simulink model "HelicopterSystem"  (R2019b)
settings: Solver=VariableStepAuto  StartTime=0.0  StopTime=10.0  RelTol=1e-3
settings Model: DataDictionary=HeliSystemDD.sldd  Creator=bpotter  LastModifiedBy=bpotter
settings DataIOCC: ExternalInput=input  LoadExternalInput=on  SaveOutput=off  DSMLogging=off  SaveTime=off  ReturnWorkspaceOutputs=off
settings OptimizationCC: UseDivisionForNetSlopeComputation=on
settings SFSimCC: CustomCodeUndefinedFunction=UseInterfaceOnly
settings ConfigComp: CovScope=ReferencedModels  CovIncludeTopModel=off

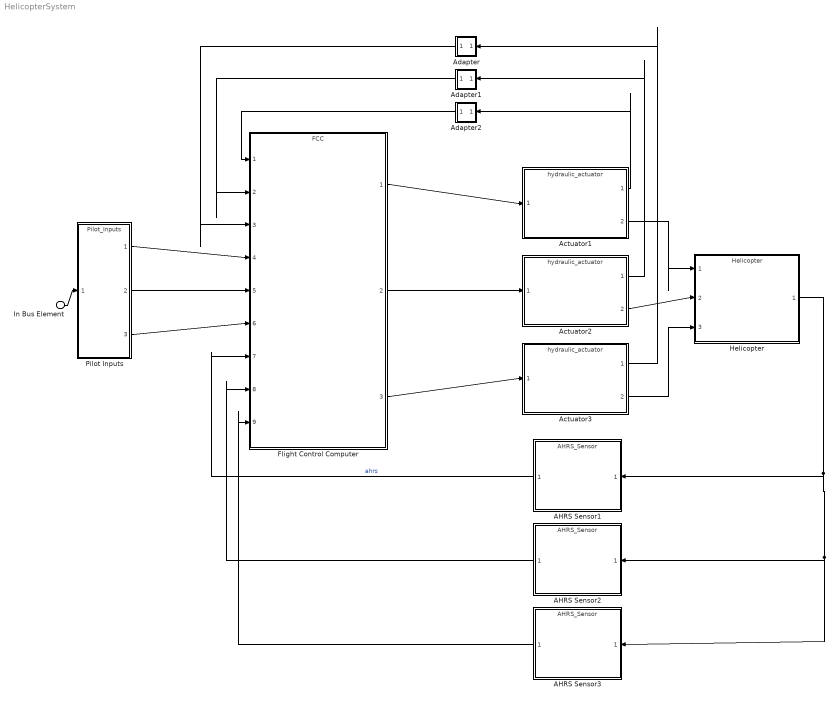
== system HelicopterSystem ==
  In Bus Element : Inport  PortName=Pilot
  "AHRS Sensor1  " : ModelReference  ModelNameDialog=AHRS_Sensor  SimulationMode=Normal  ModelReferenceVersion=1.170
      settings: PortSchema="{\"entries\":[{\"content\":{\"headerSize\":38,\"margin\":15,\"minimumSpacing\":25,\"sides\":[{\"content\":{\"connectorIds\":[\"Out1\"]},\"type\":\"ConnectorPlacement.EquallySpacedRectSide\",\"uuid\":\"b92c4a61-dac7-4e8b-978a-518464efd6dc\"},{\"content\":{\"connectorIds\":[\"In1\"],\"side\":\"RIGHT\"},\"type\":\"ConnectorPlacement.EquallySpacedRectSide\",\"uuid\":\"7fdd65f0-967d-4e66-9e23-32118f2eba6a\"},{\"content\":{\"connectorIds\":[],\"side\":\"TOP\"},\"type\":\"ConnectorPlacement.EquallySpacedRectSide\",\"uuid\":\"3746c468-edd5-479d-86e4-82fa38f92dc3\"},{\"content\":{\"connectorIds\":[],\"side\":\"BOTTOM\"},\"type\":\"ConnectorPlacement.EquallySpacedRectSide\",\"uuid\":\"6d40d3fe-09a5-49bd-a6ff-4bc99f24213d\"}]},\"type\":\"ConnectorPlacement.EquallySpacedConnector\",\"uuid\":\"540cabe7-683b-4658-aa3c-75031e0ce477\"}],\"packageUris\":[\"http:\\/\\/schema.mathworks.com\\/mf0\\/Connector\\/19700101\"],\"version\":\"1.0\"}"
  AHRS Sensor2 : ModelReference  ModelNameDialog=AHRS_Sensor  SimulationMode=Normal  ModelReferenceVersion=1.170
      settings: PortSchema="{\"entries\":[{\"content\":{\"headerSize\":38,\"margin\":15,\"minimumSpacing\":25,\"sides\":[{\"content\":{\"connectorIds\":[\"Out1\"]},\"type\":\"ConnectorPlacement.EquallySpacedRectSide\",\"uuid\":\"b92c4a61-dac7-4e8b-978a-518464efd6dc\"},{\"content\":{\"connectorIds\":[\"In1\"],\"side\":\"RIGHT\"},\"type\":\"ConnectorPlacement.EquallySpacedRectSide\",\"uuid\":\"7fdd65f0-967d-4e66-9e23-32118f2eba6a\"},{\"content\":{\"connectorIds\":[],\"side\":\"TOP\"},\"type\":\"ConnectorPlacement.EquallySpacedRectSide\",\"uuid\":\"3746c468-edd5-479d-86e4-82fa38f92dc3\"},{\"content\":{\"connectorIds\":[],\"side\":\"BOTTOM\"},\"type\":\"ConnectorPlacement.EquallySpacedRectSide\",\"uuid\":\"e1e7bc22-7c0e-4a7f-891e-467da093d39e\"}]},\"type\":\"ConnectorPlacement.EquallySpacedConnector\",\"uuid\":\"540cabe7-683b-4658-aa3c-75031e0ce477\"}],\"packageUris\":[\"http:\\/\\/schema.mathworks.com\\/mf0\\/Connector\\/19700101\"],\"version\":\"1.0\"}"
  AHRS Sensor3 : ModelReference  ModelNameDialog=AHRS_Sensor  SimulationMode=Normal  ModelReferenceVersion=1.170
      settings: PortSchema="{\"entries\":[{\"content\":{\"headerSize\":38,\"margin\":15,\"minimumSpacing\":25,\"sides\":[{\"content\":{\"connectorIds\":[\"Out1\"]},\"type\":\"ConnectorPlacement.EquallySpacedRectSide\",\"uuid\":\"b92c4a61-dac7-4e8b-978a-518464efd6dc\"},{\"content\":{\"connectorIds\":[\"In1\"],\"side\":\"RIGHT\"},\"type\":\"ConnectorPlacement.EquallySpacedRectSide\",\"uuid\":\"7fdd65f0-967d-4e66-9e23-32118f2eba6a\"},{\"content\":{\"connectorIds\":[],\"side\":\"TOP\"},\"type\":\"ConnectorPlacement.EquallySpacedRectSide\",\"uuid\":\"3746c468-edd5-479d-86e4-82fa38f92dc3\"},{\"content\":{\"connectorIds\":[],\"side\":\"BOTTOM\"},\"type\":\"ConnectorPlacement.EquallySpacedRectSide\",\"uuid\":\"265bdab0-2fd8-4d9f-89ea-736dcc13bf3d\"}]},\"type\":\"ConnectorPlacement.EquallySpacedConnector\",\"uuid\":\"540cabe7-683b-4658-aa3c-75031e0ce477\"}],\"packageUris\":[\"http:\\/\\/schema.mathworks.com\\/mf0\\/Connector\\/19700101\"],\"version\":\"1.0\"}"
  Actuator1 : ModelReference  ModelNameDialog=hydraulic_actuator  SimulationMode=Normal  ModelReferenceVersion=1.113
      settings: PortSchema="{\"entries\":[{\"content\":{\"headerSize\":38,\"margin\":15,\"minimumSpacing\":25,\"sides\":[{\"content\":{\"connectorIds\":[\"In1\"]},\"type\":\"ConnectorPlacement.EquallySpacedRectSide\",\"uuid\":\"fc9e68fb-3587-497f-b8aa-5fffad76bdc9\"},{\"content\":{\"connectorIds\":[\"Out1\",\"Out2\"],\"side\":\"RIGHT\"},\"type\":\"ConnectorPlacement.EquallySpacedRectSide\",\"uuid\":\"35b616a7-1e7e-4bab-abf4-1bdc7c33d6ef\"},{\"content\":{\"connectorIds\":[],\"side\":\"TOP\"},\"type\":\"ConnectorPlacement.EquallySpacedRectSide\",\"uuid\":\"7330c33a-79c0-425b-bf03-91b7ec739e63\"}]},\"type\":\"ConnectorPlacement.EquallySpacedConnector\",\"uuid\":\"e9501eb8-1a55-4d46-b5aa-5edf970ac40b\"}],\"packageUris\":[\"http:\\/\\/schema.mathworks.com\\/mf0\\/Connector\\/19700101\"],\"version\":\"1.0\"}"
  Actuator2 : ModelReference  ModelNameDialog=hydraulic_actuator  SimulationMode=Normal  ModelReferenceVersion=1.113
      settings: PortSchema="{\"entries\":[{\"content\":{\"headerSize\":38,\"margin\":15,\"minimumSpacing\":25,\"sides\":[{\"content\":{\"connectorIds\":[\"In1\"]},\"type\":\"ConnectorPlacement.EquallySpacedRectSide\",\"uuid\":\"fc9e68fb-3587-497f-b8aa-5fffad76bdc9\"},{\"content\":{\"connectorIds\":[\"Out1\",\"Out2\"],\"side\":\"RIGHT\"},\"type\":\"ConnectorPlacement.EquallySpacedRectSide\",\"uuid\":\"35b616a7-1e7e-4bab-abf4-1bdc7c33d6ef\"},{\"content\":{\"connectorIds\":[],\"side\":\"TOP\"},\"type\":\"ConnectorPlacement.EquallySpacedRectSide\",\"uuid\":\"7330c33a-79c0-425b-bf03-91b7ec739e63\"}]},\"type\":\"ConnectorPlacement.EquallySpacedConnector\",\"uuid\":\"e9501eb8-1a55-4d46-b5aa-5edf970ac40b\"}],\"packageUris\":[\"http:\\/\\/schema.mathworks.com\\/mf0\\/Connector\\/19700101\"],\"version\":\"1.0\"}"
  Actuator3 : ModelReference  ModelNameDialog=hydraulic_actuator  SimulationMode=Normal  ModelReferenceVersion=1.113
      settings: PortSchema="{\"entries\":[{\"content\":{\"headerSize\":38,\"margin\":15,\"minimumSpacing\":25,\"sides\":[{\"content\":{\"connectorIds\":[\"In1\"]},\"type\":\"ConnectorPlacement.EquallySpacedRectSide\",\"uuid\":\"fc9e68fb-3587-497f-b8aa-5fffad76bdc9\"},{\"content\":{\"connectorIds\":[\"Out1\",\"Out2\"],\"side\":\"RIGHT\"},\"type\":\"ConnectorPlacement.EquallySpacedRectSide\",\"uuid\":\"35b616a7-1e7e-4bab-abf4-1bdc7c33d6ef\"},{\"content\":{\"connectorIds\":[],\"side\":\"TOP\"},\"type\":\"ConnectorPlacement.EquallySpacedRectSide\",\"uuid\":\"7330c33a-79c0-425b-bf03-91b7ec739e63\"}]},\"type\":\"ConnectorPlacement.EquallySpacedConnector\",\"uuid\":\"e9501eb8-1a55-4d46-b5aa-5edf970ac40b\"}],\"packageUris\":[\"http:\\/\\/schema.mathworks.com\\/mf0\\/Connector\\/19700101\"],\"version\":\"1.0\"}"
  Adapter : Subsystem
      settings: PortSchema="{\"entries\":[{\"content\":{\"margin\":10,\"minimumSpacing\":10,\"sides\":[{\"content\":{\"connectorIds\":[\"Out1\"]},\"type\":\"ConnectorPlacement.EquallySpacedRectSide\",\"uuid\":\"3ae78bc2-40c3-4405-b1e9-aa99f01667e3\"},{\"content\":{\"connectorIds\":[\"In1\"],\"side\":\"RIGHT\"},\"type\":\"ConnectorPlacement.EquallySpacedRectSide\",\"uuid\":\"ba8b0a16-3184-49c7-8dc0-2ecd07e7bfdb\"},{\"content\":{\"connectorIds\":[],\"side\":\"TOP\"},\"type\":\"ConnectorPlacement.EquallySpacedRectSide\",\"uuid\":\"2e1b4a4d-beaa-4cad-b3d0-913db021f2bf\"},{\"content\":{\"connectorIds\":[],\"side\":\"BOTTOM\"},\"type\":\"ConnectorPlacement.EquallySpacedRectSide\",\"uuid\":\"ce88d55a-ed5b-4e72-9847-8844dc7d3e9c\"}]},\"type\":\"ConnectorPlacement.EquallySpacedConnector\",\"uuid\":\"3893b0a5-5763-428c-b0ac-b513abbdb3d9\"}],\"packageUris\":[\"http://schema.mathworks.com/mf0/Connector/19700101\"],\"version\":\"1.0\"}"
  Adapter1 : Subsystem
      settings: PortSchema="{\"entries\":[{\"content\":{\"margin\":10,\"minimumSpacing\":10,\"sides\":[{\"content\":{\"connectorIds\":[\"Out1\"]},\"type\":\"ConnectorPlacement.EquallySpacedRectSide\",\"uuid\":\"3ae78bc2-40c3-4405-b1e9-aa99f01667e3\"},{\"content\":{\"connectorIds\":[\"In1\"],\"side\":\"RIGHT\"},\"type\":\"ConnectorPlacement.EquallySpacedRectSide\",\"uuid\":\"ba8b0a16-3184-49c7-8dc0-2ecd07e7bfdb\"},{\"content\":{\"connectorIds\":[],\"side\":\"TOP\"},\"type\":\"ConnectorPlacement.EquallySpacedRectSide\",\"uuid\":\"2e1b4a4d-beaa-4cad-b3d0-913db021f2bf\"},{\"content\":{\"connectorIds\":[],\"side\":\"BOTTOM\"},\"type\":\"ConnectorPlacement.EquallySpacedRectSide\",\"uuid\":\"ce88d55a-ed5b-4e72-9847-8844dc7d3e9c\"}]},\"type\":\"ConnectorPlacement.EquallySpacedConnector\",\"uuid\":\"3893b0a5-5763-428c-b0ac-b513abbdb3d9\"}],\"packageUris\":[\"http://schema.mathworks.com/mf0/Connector/19700101\"],\"version\":\"1.0\"}"
  Adapter2 : Subsystem
      settings: PortSchema="{\"entries\":[{\"content\":{\"margin\":10,\"minimumSpacing\":10,\"sides\":[{\"content\":{\"connectorIds\":[\"Out1\"]},\"type\":\"ConnectorPlacement.EquallySpacedRectSide\",\"uuid\":\"3ae78bc2-40c3-4405-b1e9-aa99f01667e3\"},{\"content\":{\"connectorIds\":[\"In1\"],\"side\":\"RIGHT\"},\"type\":\"ConnectorPlacement.EquallySpacedRectSide\",\"uuid\":\"ba8b0a16-3184-49c7-8dc0-2ecd07e7bfdb\"},{\"content\":{\"connectorIds\":[],\"side\":\"TOP\"},\"type\":\"ConnectorPlacement.EquallySpacedRectSide\",\"uuid\":\"2e1b4a4d-beaa-4cad-b3d0-913db021f2bf\"},{\"content\":{\"connectorIds\":[],\"side\":\"BOTTOM\"},\"type\":\"ConnectorPlacement.EquallySpacedRectSide\",\"uuid\":\"ce88d55a-ed5b-4e72-9847-8844dc7d3e9c\"}]},\"type\":\"ConnectorPlacement.EquallySpacedConnector\",\"uuid\":\"3893b0a5-5763-428c-b0ac-b513abbdb3d9\"}],\"packageUris\":[\"http://schema.mathworks.com/mf0/Connector/19700101\"],\"version\":\"1.0\"}"
  Flight Control Computer : ModelReference  ModelNameDialog=FCC  SimulationMode=Normal  ModelReferenceVersion=1.70
      settings: PortSchema="{\"entries\":[{\"content\":{\"headerSize\":38,\"margin\":15,\"minimumSpacing\":25,\"sides\":[{\"content\":{\"connectorIds\":[\"In1\",\"In2\",\"In3\",\"In4\",\"In5\",\"In6\",\"In7\",\"In8\",\"In9\"]},\"type\":\"ConnectorPlacement.EquallySpacedRectSide\",\"uuid\":\"9959663a-a09f-47a8-9233-f49ef842a145\"},{\"content\":{\"connectorIds\":[\"Out1\",\"Out2\",\"Out3\"],\"side\":\"RIGHT\"},\"type\":\"ConnectorPlacement.EquallySpacedRectSide\",\"uuid\":\"4d21989f-a787-4fcb-862b-70f89eaf4b18\"},{\"content\":{\"connectorIds\":[],\"side\":\"TOP\"},\"type\":\"ConnectorPlacement.EquallySpacedRectSide\",\"uuid\":\"c2e05887-1556-4bab-9344-e41638b7e6c9\"}]},\"type\":\"ConnectorPlacement.EquallySpacedConnector\",\"uuid\":\"3e276280-9190-46ce-8e07-322db49b607e\"}],\"packageUris\":[\"http:\\/\\/schema.mathworks.com\\/mf0\\/Connector\\/19700101\"],\"version\":\"1.0\"}"
  Helicopter : ModelReference  ModelNameDialog=Helicopter  SimulationMode=Normal  ModelReferenceVersion=1.168
      settings: PortSchema="{\"entries\":[{\"content\":{\"headerSize\":38,\"margin\":15,\"minimumSpacing\":25,\"sides\":[{\"content\":{\"connectorIds\":[\"In1\",\"In2\",\"In3\"]},\"type\":\"ConnectorPlacement.EquallySpacedRectSide\",\"uuid\":\"b92c4a61-dac7-4e8b-978a-518464efd6dc\"},{\"content\":{\"connectorIds\":[\"Out1\"],\"side\":\"RIGHT\"},\"type\":\"ConnectorPlacement.EquallySpacedRectSide\",\"uuid\":\"7fdd65f0-967d-4e66-9e23-32118f2eba6a\"},{\"content\":{\"connectorIds\":[],\"side\":\"TOP\"},\"type\":\"ConnectorPlacement.EquallySpacedRectSide\",\"uuid\":\"3746c468-edd5-479d-86e4-82fa38f92dc3\"}]},\"type\":\"ConnectorPlacement.EquallySpacedConnector\",\"uuid\":\"540cabe7-683b-4658-aa3c-75031e0ce477\"}],\"packageUris\":[\"http:\\/\\/schema.mathworks.com\\/mf0\\/Connector\\/19700101\"],\"version\":\"1.0\"}"
  Pilot Inputs : ModelReference  ModelNameDialog=Pilot_Inputs  SimulationMode=Normal  ModelReferenceVersion=1.169
      settings: PortSchema="{\"entries\":[{\"content\":{\"headerSize\":38,\"margin\":15,\"minimumSpacing\":25,\"sides\":[{\"content\":{\"connectorIds\":[\"In1\"]},\"type\":\"ConnectorPlacement.EquallySpacedRectSide\",\"uuid\":\"c30acc98-d6f3-4b20-b0da-834679cd871f\"},{\"content\":{\"connectorIds\":[\"Out1\",\"Out2\",\"Out3\"],\"side\":\"RIGHT\"},\"type\":\"ConnectorPlacement.EquallySpacedRectSide\",\"uuid\":\"00258b73-8db9-4b2a-9802-819ef35b883c\"},{\"content\":{\"connectorIds\":[],\"side\":\"TOP\"},\"type\":\"ConnectorPlacement.EquallySpacedRectSide\",\"uuid\":\"0c08f240-221e-4cf9-aab1-bb2491e3d13f\"}]},\"type\":\"ConnectorPlacement.EquallySpacedConnector\",\"uuid\":\"936bca2f-e841-45ae-81c4-5f1a94e8ce36\"}],\"packageUris\":[\"http:\\/\\/schema.mathworks.com\\/mf0\\/Connector\\/19700101\"],\"version\":\"1.0\"}"
  wires:
  Flight Control Computer/1 -> Actuator1/1
  Flight Control Computer/2 -> Actuator2/1
  Flight Control Computer/3 -> Actuator3/1
  Pilot Inputs/1 -> Flight Control Computer/4
  Pilot Inputs/2 -> Flight Control Computer/5
  Pilot Inputs/3 -> Flight Control Computer/6
  Actuator2/2 -> Helicopter/2
  Actuator1/2 -> Helicopter/1
  Actuator3/2 -> Helicopter/3
  Helicopter/1 -> AHRS Sensor3/1, AHRS Sensor2/1, "AHRS Sensor1  "/1
  "AHRS Sensor1  "/1 -> Flight Control Computer/7  "ahrs"
  AHRS Sensor2/1 -> Flight Control Computer/8
  AHRS Sensor3/1 -> Flight Control Computer/9
  Actuator1/1 -> Adapter2/1(In)
  Adapter2/1(Out) -> Flight Control Computer/1
  Actuator2/1 -> Adapter1/1(In)
  Adapter1/1(Out) -> Flight Control Computer/2
  Adapter/1(Out) -> Flight Control Computer/3
  Actuator3/1 -> Adapter/1(In)
  In Bus Element/1 -> Pilot Inputs/1

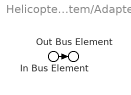
== system HelicopterSystem/Adapter ==
  In Bus Element : Inport  PortName=In
  Out Bus Element : Outport  PortName=Out
  wires:
  In Bus Element/1 -> Out Bus Element/1

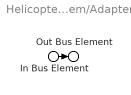
== system HelicopterSystem/Adapter1 ==
  In Bus Element : Inport  PortName=In
  Out Bus Element : Outport  PortName=Out
  wires:
  In Bus Element/1 -> Out Bus Element/1

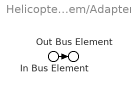
== system HelicopterSystem/Adapter2 ==
  In Bus Element : Inport  PortName=In
  Out Bus Element : Outport  PortName=Out
  wires:
  In Bus Element/1 -> Out Bus Element/1
